simulink model "system2"  (R2019b)
settings: Solver=VariableStepAuto  StartTime=0.0  StopTime=15  RelTol=1e-5
Description:
  | 高阶系统闭环主导极点分析
settings Model: Creator=Inspiron  LastModifiedBy=Inspiron

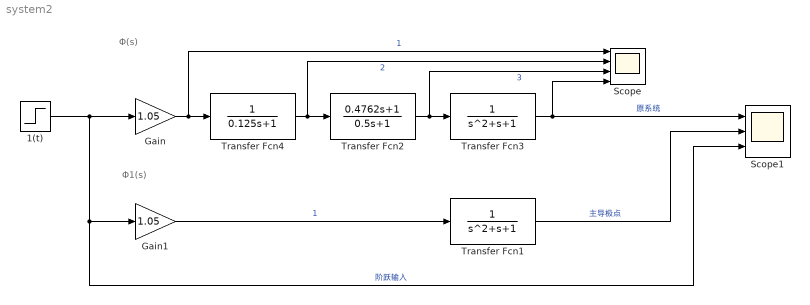
== system system2 ==
  note: Φ(s)
  note: Φ1(s)
  1(t) : Step  SampleTime=0
  Gain : Gain  Gain=1.05
  Gain1 : Gain  Gain=1.05
  Scope : Scope  NumInputPorts=4
  Scope1 : Scope  NumInputPorts=3
  Transfer Fcn1 : TransferFcn  Denominator=[1 1 1]
  Transfer Fcn2 : TransferFcn  Numerator=[0.4762 1]  Denominator=[0.5 1]
  Transfer Fcn3 : TransferFcn  Denominator=[1 1 1]
  Transfer Fcn4 : TransferFcn  Denominator=[0.125 1]
  wires:
  Transfer Fcn1/1 -> Scope1/2  "主导极点"
  Gain1/1 -> Transfer Fcn1/1  "1"
  Transfer Fcn3/1 -> Scope1/1, Scope/4  "原系统"
  1(t)/1 -> Gain1/1, Scope1/3, Gain/1  "阶跃输入"
  Transfer Fcn2/1 -> Scope/3, Transfer Fcn3/1  "3"
  Transfer Fcn4/1 -> Scope/2, Transfer Fcn2/1  "2"
  Gain/1 -> Scope/1, Transfer Fcn4/1  "1"
